simulink model "template_seesaw_2021b"  (R2021b)
settings: Solver=FixedStepDiscrete  StartTime=0.0  StopTime=inf  FixedStep=0.005  RelTol=1e-3
values from neighbouring files (symbols this model uses):
  alfa = omega_c*Ts/(1+omega_c*Ts)    (= 0.0591173974417)    [closed_loop2.m]
  beta = omega_c2*Ts/(1+omega_c2*Ts)    (= 0.135755248164)    [closed_loop2.m]
  K = lqr(A,B,Q,R)    [closed_loop1.m]
  Ts = 0.005    [closed_loop2.m]
undefined symbols (not defined in the file or in its folder): National_Instruments, PCI
libraries: sldrtlib x2, simulink_extras x1
settings Model: SimulationMode=external  ExtModeTrigDuration=200000  Creator=magudelo  LastModifiedBy=pieter
settings SolverCC: AlgebraicLoopSolver=TrustRegion  InsertRTBMode=Always
settings DataIOCC: LimitDataPoints=on  SaveFormat=Array  SignalLoggingSaveFormat=ModelDataLogs  ReturnWorkspaceOutputs=off
settings OptimizationCC: ExpressionDepthLimit=2147483647
settings DebuggingCC: UnderspecifiedInitializationDetection=Classic  MergeDetectMultiDrivingBlocksExec=none  SolverPrmCheckMsg=warning  FcnCallInpInsideContextMsg=warning  StateNameClashWarn=warning  PregeneratedLibrarySubsystemCodeDiagnostic=none  SFUnexpectedBacktrackingDiag=warning  SFNoUnconditionalDefaultTransitionDiag=warning  SFExecutionAtInitializationDiag=none  SFMachineParentedDataDiag=warning  ArithmeticOperatorsInVariantConditions=warning
settings ModelReferenceCC: PropagateSignalLabelsOutOfModel=off
settings SFSimCC: SimUseLocalCustomCode=off  CustomCodeUndefinedFunction=UseInterfaceOnly
settings RTWCC: Description=Simulink Desktop Real-Time  SystemTargetFile=sldrt.tlc  TemplateMakefile=sldrt.tmf  RTWUseLocalCustomCode=off  RTWCompilerOptimization=on
settings CodeAppCC: MaxIdLength=95  StateflowObjectComments=on
settings SimulinkDesktopRealTimeCC: TargetPreCompLibLocation=C:\Program Files\MATLAB\R2021b\toolbox\sldrt\lib\win64  TargetLangStandard=C89/C90 (ANSI)  SupportVariableSizeSignals=off
settings ConfigComp: CovMetricSettings=dw  CovSaveCumulativeToWorkspaceVar=on  CovSaveSingleToWorkspaceVar=on  CovExternalEMLEnable=off

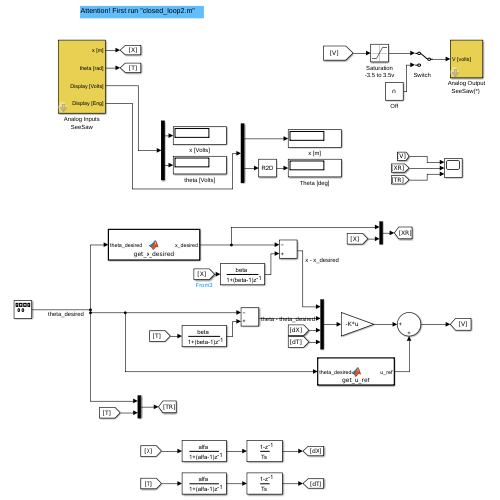
[thumbnail: Simulink's stored preview of the top-level diagram]
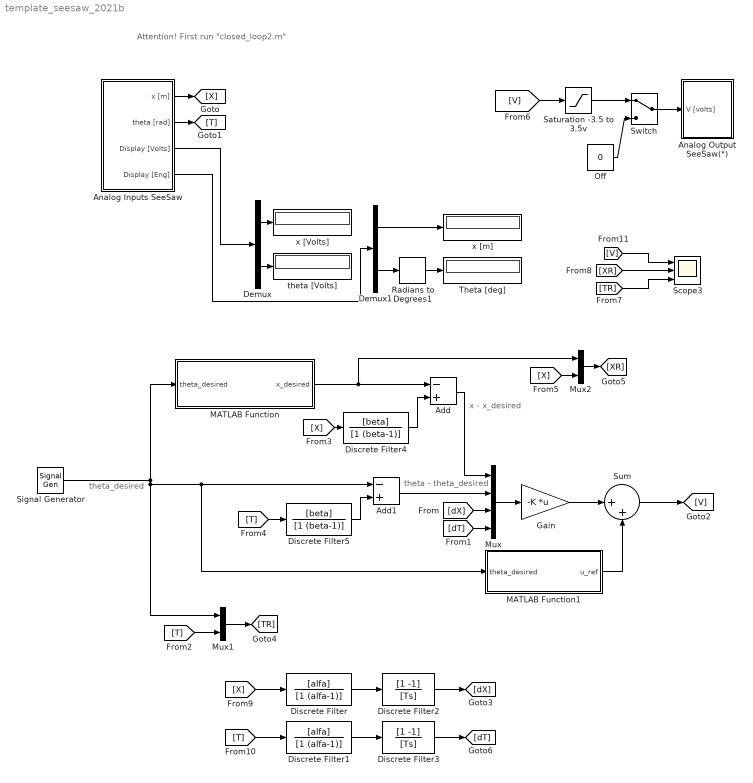
== system template_seesaw_2021b ==
  note: Attention! First run "closed_loop2.m"
  note: x - x_desired
  note: theta_desired
  note: theta - theta_desired
  Add : Sum  Inputs=-+
  Add1 : Sum  Inputs=-+
  Analog Inputs SeeSaw : Subsystem  mask(Analog Inputs. SeeSaw){v2m=0.1033, offset_x=0, v2r=-0.0827, offset_theta=-5.56}
      mask prompts: v2m "F_x = Conversion factor from Volts to Meters:"; offset_x "Off_x = Offset for Cart Position [Volts] :"; v2r "F_theta = Conversion Factor From Volts to Radians :"; offset_theta "Off_theta = Offset for the angle of the SeeSaw [Volts] :"
      mask help:
      | Remember:
      |    Cart Position (x)                     => channel ACH0
      |    Angle of the SeeSaw (theta) => channel ACH1
      |
      |   Cart Position [m] = F_x *  ( Cart Position [v] + off_x )
      |   Angle of the SeeSaw [rad] = F_theta *  ( Angle of the SeeSaw [v] + off_theta )
  "Analog Output SeeSaw(*) " : Subsystem  mask(Analog Output - SeeSaw){}
      mask help:
      | Remember
      |    AO 0 => Power Amplifier + Motor
  Demux : Demux  Outputs=2
  Demux1 : Demux  Outputs=2
  Discrete Filter : DiscreteFilter  Numerator=[alfa]  Denominator=[1 (alfa-1)]
  Discrete Filter1 : DiscreteFilter  Numerator=[alfa]  Denominator=[1 (alfa-1)]
  Discrete Filter2 : DiscreteFilter  Numerator=[1 -1]  Denominator=[Ts]
  Discrete Filter3 : DiscreteFilter  Numerator=[1 -1]  Denominator=[Ts]
  Discrete Filter4 : DiscreteFilter  Numerator=[beta]  Denominator=[1 (beta-1)]
  Discrete Filter5 : DiscreteFilter  Numerator=[beta]  Denominator=[1 (beta-1)]
  Gain : Gain  Gain=-K  Multiplication=Matrix(K*u)
  MATLAB Function : MATLAB Function  TreatAsAtomicUnit=on
  MATLAB Function1 : MATLAB Function  TreatAsAtomicUnit=on
  Mux : Mux
  Mux1 : Mux  Inputs=2
  Mux2 : Mux  Inputs=2
  Off : Constant  Value=0
  Radians to Degrees1 : simulink_extras/Transformations/Radians to Degrees
  Saturation -3.5 to 3.5v : Saturate  UpperLimit=3.5  LowerLimit=-3.5
  Scope3 : Scope  NumInputPorts=3
  Signal Generator : SignalGenerator  WaveForm=square  Amplitude=pi/180*5  Frequency=.10
  Sum : Sum  Inputs=|++
  "Switch  " : ManualSwitch
  Theta [deg] : Display
      settings: SampleTime=0.25
  theta [Volts] : Display
      settings: SampleTime=0.25
  x [Volts] : Display
      settings: SampleTime=0.25
  x [m] : Display
      settings: SampleTime=0.25
  wires:
  Demux/1 -> x [Volts]/1
  Demux/2 -> theta [Volts]/1
  Analog Inputs SeeSaw/3(Display [Volts]) -> Demux/1
  Analog Inputs SeeSaw/4(Display [Eng]) -> Demux1/1
  Off/1 -> "Switch  "/2
  "Switch  "/1 -> "Analog Output SeeSaw(*) "/1(V [volts])
  Demux1/1 -> x [m]/1
  Demux1/2 -> Radians to Degrees1/1
  Radians to Degrees1/1 -> Theta [deg]/1
  Saturation -3.5 to 3.5v/1 -> "Switch  "/1
  Analog Inputs SeeSaw/2(theta [rad]) -> [T]
  Analog Inputs SeeSaw/1(x [m]) -> [X]
  Add/1 -> Mux/1
  Discrete Filter5/1 -> Add1/2
  [dX] -> Mux/3
  MATLAB Function1/1(u_ref) -> Sum/2
  Add1/1 -> Mux/2
  Discrete Filter4/1 -> Add/2
  [T] -> Discrete Filter5/1
  [X] -> Discrete Filter4/1
  [dT] -> Mux/4
  Signal Generator/1 -> Mux1/1, MATLAB Function1/1(theta_desired), Add1/1, MATLAB Function/1(theta_desired)
  Gain/1 -> Sum/1
  Mux/1 -> Gain/1
  MATLAB Function/1(x_desired) -> Mux2/1, Add/1
  Mux2/1 -> [XR]
  [T] -> Mux1/2
  Mux1/1 -> [TR]
  [X] -> Mux2/2
  Sum/1 -> [V]
  [V] -> Saturation -3.5 to 3.5v/1
  [T] -> Discrete Filter1/1
  [X] -> Discrete Filter/1
  Discrete Filter/1 -> Discrete Filter2/1
  Discrete Filter1/1 -> Discrete Filter3/1
  Discrete Filter3/1 -> [dT]
  Discrete Filter2/1 -> [dX]
  [XR] -> Scope3/2
  [V] -> Scope3/1
  [TR] -> Scope3/3

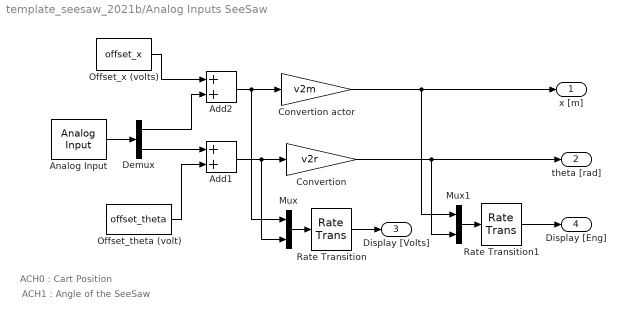
== system template_seesaw_2021b/Analog Inputs SeeSaw ==
  note: ACH0 : Cart Position
  note: ACH1 : Angle of the SeeSaw
  Add1 : Sum
  Add2 : Sum
  Analog Input : sldrtlib/Analog Input  SampleTime=0.005  MaxMissedTicks=10  ShowMissedTicks=off  YieldWhenWaiting=off  DrvName=National_Instruments/PCI-6014  DrvAddress=4294967295  DrvOptions=[1 0 0 0 0 0]  Channels=[1 2]  RangeMode=1  VoltRange=1  DataType=1
      settings: AttributesFormatString=National Instruments\nPCI-6014 [auto]
  "Convertion " : Gain  Gain=v2r
  Convertion actor : Gain  Gain=v2m
  Demux : Demux  Outputs=2
  Mux : Mux  Inputs=2
  Mux1 : Mux  Inputs=2
  Offset_theta (volt) : Constant  Value=offset_theta
  Offset_x (volts) : Constant  Value=offset_x
  Rate Transition : RateTransition  OutPortSampleTime=0.25
  Rate Transition1 : RateTransition  OutPortSampleTime=0.25
  x [m] : Outport  VectorParamsAs1DForOutWhenUnconnected=off
  theta [rad] : Outport  Port=2  VectorParamsAs1DForOutWhenUnconnected=off
  Display [Volts] : Outport  Port=3  VectorParamsAs1DForOutWhenUnconnected=off
  Display [Eng] : Outport  Port=4  VectorParamsAs1DForOutWhenUnconnected=off
  wires:
  Analog Input/1 -> Demux/1
  Demux/1 -> Add2/2
  Add2/1 -> Convertion actor/1, Mux/1
  Offset_x (volts)/1 -> Add2/1
  Convertion actor/1 -> x [m]/1, Mux1/1
  Demux/2 -> Add1/1
  Offset_theta (volt)/1 -> Add1/2
  Add1/1 -> "Convertion "/1, Mux/2
  "Convertion "/1 -> theta [rad]/1, Mux1/2
  Rate Transition/1 -> Display [Volts]/1
  Mux/1 -> Rate Transition/1
  Mux1/1 -> Rate Transition1/1
  Rate Transition1/1 -> Display [Eng]/1

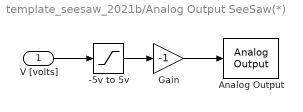
== system template_seesaw_2021b/Analog Output SeeSaw(*)  ==
  V [volts] : Inport
  -5v to 5v : Saturate  UpperLimit=5  LowerLimit=-5
  Analog Output : sldrtlib/Analog Output  SampleTime=0.005  MaxMissedTicks=10  ShowMissedTicks=off  YieldWhenWaiting=off  DrvName=National_Instruments/PCI-6014  DrvAddress=4294967295  DrvOptions=[1 0 0 0 0 0]  Channels=1  RangeMode=1  VoltRange=1  InitialValue=0  FinalValue=0
      settings: AttributesFormatString=National Instruments\nPCI-6014 [auto]
  Gain : Gain  Gain=-1
  wires:
  Gain/1 -> Analog Output/1
  -5v to 5v/1 -> Gain/1
  V [volts]/1 -> -5v to 5v/1

== matlab function template_seesaw_2021b/MATLAB Function ==
  data: theta_desired input; x_desired output
function x_desired = get_x_desired(theta_desired)
    Mc = 0.52;
    Msw = 3.6;
    Dt = 0.1250;
    Dc = 0.058;
    % From equation (13)
    x_desired = (Mc*Dt+Msw*Dc)*tan(theta_desired)/Mc;
end

== matlab function template_seesaw_2021b/MATLAB Function1 ==
  data: theta_desired input; u_ref output
function u_ref = get_u_ref(theta_desired)
Mc = 0.52;
g = 9.81;
F = Mc*g*sin(theta_desired);
Kt = 0.00767;
Kg = 3.71;
eta_m = 1;
eta_g = 1;
Rm = 2.6;
r = 0.00635;
u_ref = Rm*r/(eta_m*eta_g*Kt*Kg)*F;
